simulink model "smc_mass_1d"  (R2018a)
settings: Solver=ode4  StartTime=0.0  StopTime=20.0  FixedStep=ts  RelTol=1e-3
values from neighbouring files (symbols this model uses):
  B = 0    [run_simu.m]
  M = 1    [run_simu.m]
libraries: simulink x2
settings Model: Creator=auralius  LastModifiedBy=Yimin Zhao
settings DataIOCC: LimitDataPoints=on  SaveFormat=Array
settings OptimizationCC: BlockReduction=off  BooleanDataType=off  LifeSpan=inf
settings DebuggingCC: SaveWithParameterizedLinksMsg=none  UnderspecifiedInitializationDetection=Classic  MergeDetectMultiDrivingBlocksExec=none  SignalResolutionControl=TryResolveAllWithWarning  SFUnexpectedBacktrackingDiag=warning  SFNoUnconditionalDefaultTransitionDiag=warning  SFExecutionAtInitializationDiag=none
settings HardwareCC: ProdBitPerPointer=32  ProdBitPerSizeT=32  ProdBitPerPtrDiffT=32  ProdLargestAtomicFloat=None  ProdIntDivRoundTo=Undefined  ProdEndianess=Unspecified  ProdWordSize=32  ProdHWDeviceType=32-bit Generic  TargetUnknown=on
settings ModelReferenceCC: PropagateSignalLabelsOutOfModel=off
settings CodeAppCC: StateflowObjectComments=on
settings GRTTargetCC: TargetLangStandard=C89/C90 (ANSI)  GeneratePreprocessorConditionals=Disable all
settings ConfigComp: CovMetricSettings=dw  CovHtmlReporting=on  CovSaveCumulativeToWorkspaceVar=on  CovSaveSingleToWorkspaceVar=on  CovExternalEMLEnable=off

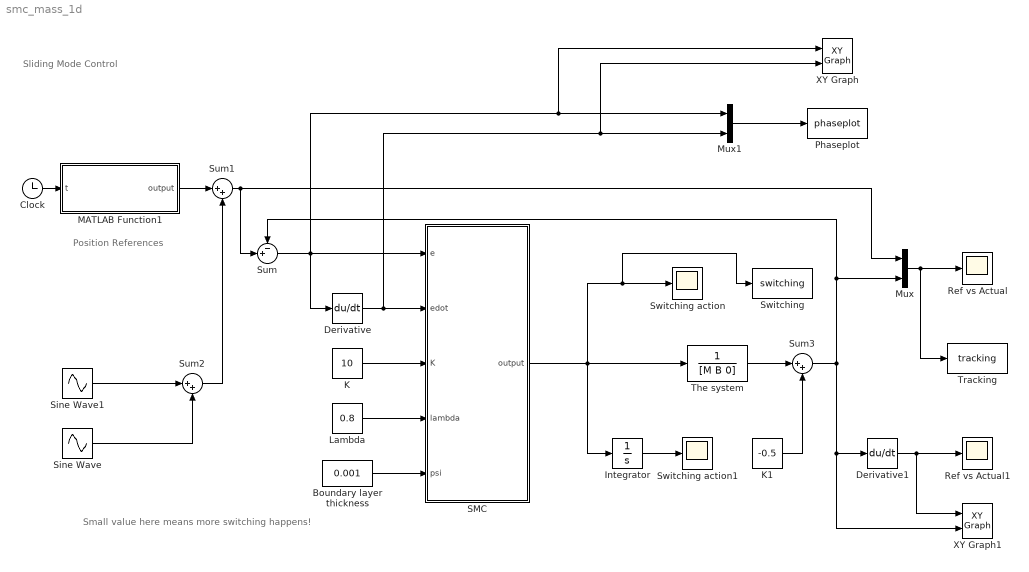
== system smc_mass_1d ==
  note: Small value here means more switching happens!
  note: Sliding Mode Control
  note: Position References
  Boundary layer thickness : Constant  Value=0.001
  Clock : Clock
  Derivative : Derivative
  Derivative1 : Derivative
  Integrator : Integrator
  K : Constant  Value=10
  K1 : Constant  Value=-0.5
  Lambda : Constant  Value=0.8
  MATLAB Function1 : MATLAB Function  TreatAsAtomicUnit=on
  Mux : Mux  Inputs=2
  Mux1 : Mux  Inputs=2
  Phaseplot : ToWorkspace  VariableName=phaseplot  SampleTime=-1
  Ref vs Actual : Scope
  Ref vs Actual1 : Scope
  SMC : MATLAB Function  TreatAsAtomicUnit=on
  Sine Wave : Sin  SampleTime=0
  Sine Wave1 : Sin  Amplitude=0.2  Frequency=0.2  SampleTime=0
  Sum : Sum  Inputs=-+|
  Sum1 : Sum  Inputs=|++
  Sum2 : Sum  Inputs=|++
  Sum3 : Sum  Inputs=|++
  Switching : ToWorkspace  VariableName=switching  SampleTime=-1
  Switching action : Scope
  Switching action1 : Scope
  The system : TransferFcn  Denominator=[M B 0]
  Tracking : ToWorkspace  VariableName=tracking  SampleTime=-1
  XY Graph : simulink/Sinks/XY Graph  xmin=-1  xmax=2  ymin=-1  ymax=2  st=-1
  XY Graph1 : simulink/Sinks/XY Graph  xmin=-2  xmax=2  ymin=-2  ymax=2  st=-1
  wires:
  Derivative/1 -> XY Graph/2, Mux1/2, SMC/2(edot)
  Sum/1 -> XY Graph/1, Mux1/1, SMC/1(e), Derivative/1
  Lambda/1 -> SMC/4(lambda)
  K/1 -> SMC/3(K)
  Boundary layer thickness/1 -> SMC/5(psi)
  Mux/1 -> Tracking/1, Ref vs Actual/1
  SMC/1(output) -> Integrator/1, The system/1, Switching/1, Switching action/1
  MATLAB Function1/1(output) -> Sum1/1
  Clock/1 -> MATLAB Function1/1(t)
  Mux1/1 -> Phaseplot/1
  Sine Wave/1 -> Sum2/2
  Sine Wave1/1 -> Sum2/1
  Sum2/1 -> Sum1/2
  Sum1/1 -> Mux/1, Sum/2
  Derivative1/1 -> XY Graph1/1, Ref vs Actual1/1
  Integrator/1 -> Switching action1/1
  The system/1 -> Sum3/1
  Sum3/1 -> XY Graph1/2, Derivative1/1, Mux/2, Sum/1
  K1/1 -> Sum3/2

== matlab function smc_mass_1d/SMC ==
  data: e input; output output; edot input; K input; lambda input; psi input
function output = smc(e, edot, K, lambda, psi)
%#codegen

    s = lambda * e + edot;
        
    if (abs(s) > psi)    
        sat_s = sign(s);
    else
        sat_s = s/psi;
    end
    
    output = -(edot - K * sat_s);

end

== matlab function smc_mass_1d/MATLAB Function1 ==
  data: t input; output output
function output = generate_input(t)
%#codegen

    %output = -pi/2+52.5/180*pi*(1-cos(1.26*t));
    output = cos(1.26*t);
    
end
